simulink model "AGTF30SysLin"  (Simulink 8.5)
settings: Solver=FixedStepDiscrete  StartTime=0.0  StopTime=MWS.In.Max_IterSS  FixedStep=1  RelTol=1e-3
undefined symbols (not defined in the file or in its folder): MWS
libraries: Lib_Cntrl_SetPoint_TMATS x2, Lib_Solve_IterNRSolverJC_TMATS x1, Lib_Solve_Linearize_TMATS x1
settings Model: Creator=jwchapm2  LastModifiedBy=jwchapm2
settings DataIOCC: SignalLoggingSaveFormat=Dataset
settings OptimizationCC: ExpressionDepthLimit=128
settings DebuggingCC: UnderspecifiedInitializationDetection=Simplified  MergeDetectMultiDrivingBlocksExec=error  FcnCallInpInsideContextMsg=EnableAllAsError  StateNameClashWarn=none
settings GRTTargetCC: CombineOutputUpdateFcns=on  GRTInterface=off

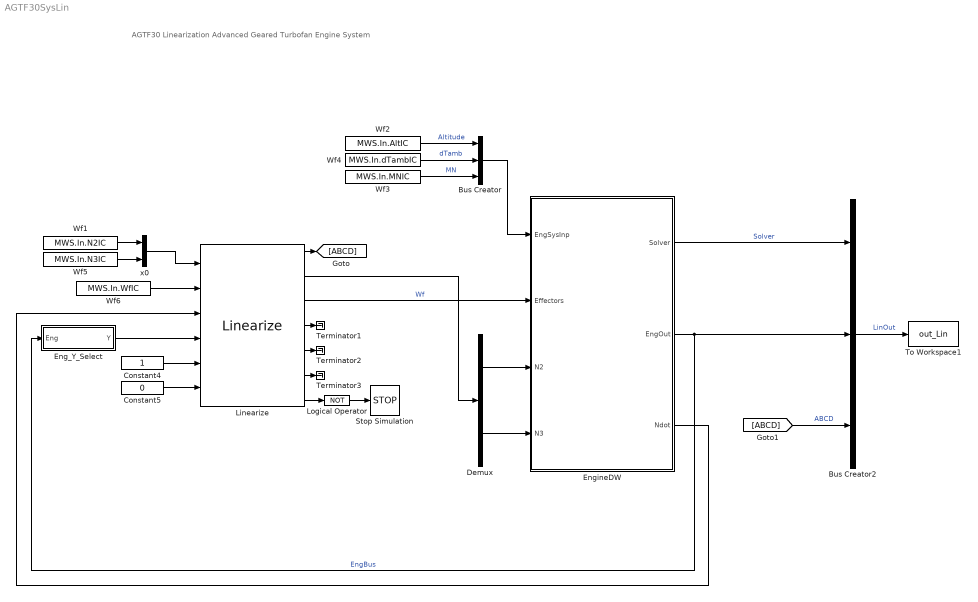
== system AGTF30SysLin ==
  note: AGTF30 Linearization
      | Advanced Geared Turbofan Engine System
  Bus Creator : BusCreator  Inputs=3
  Bus Creator2 : BusCreator  Inputs=3
  Constant4 : Constant
  Constant5 : Constant  Value=0
  Demux : Demux  Outputs=2
  Eng_Y_Select : Subsystem
  EngineDW : Subsystem
  Linearize : Lib_Solve_Linearize_TMATS/Linearize  N_XPer_M=MWS.In.XPerLin  N_UPer_M=MWS.In.UPerLin  N_Y_M=8
  Logical Operator : Logic  Operator=NOT  AllPortsSameDT=off  OutDataTypeStr=boolean
  Stop Simulation : Stop
  Terminator1 : Terminator
  Terminator2 : Terminator
  Terminator3 : Terminator
  To Workspace1 : ToWorkspace  VariableName=out_Lin  SaveFormat=Timeseries  SampleTime=-1
      settings: MaxDataPoints=1
  Wf1 : Constant  Value=MWS.In.N2IC
  Wf2 : Constant  Value=MWS.In.AltIC
  Wf3 : Constant  Value=MWS.In.MNIC
  Wf4 : Constant  Value=MWS.In.dTambIC
  Wf5 : Constant  Value=MWS.In.N3IC
  Wf6 : Constant  Value=MWS.In.WfIC
  x0 : Mux  Inputs=2
  wires:
  Wf2/1 -> Bus Creator/1  "Altitude"
  Wf4/1 -> Bus Creator/2  "dTamb"
  Wf3/1 -> Bus Creator/3  "MN"
  Bus Creator/1 -> EngineDW/1(EngSysInp)
  Demux/1 -> EngineDW/3(N2)
  Demux/2 -> EngineDW/4(N3)
  Linearize/2 -> Demux/1
  Linearize/3 -> EngineDW/2(Effectors)  "Wf"
  Linearize/4 -> Terminator1/1
  Linearize/5 -> Terminator2/1
  Linearize/6 -> Terminator3/1
  Logical Operator/1 -> Stop Simulation/1
  Linearize/7 -> Logical Operator/1
  Constant4/1 -> Linearize/5
  Constant5/1 -> Linearize/6
  Wf1/1 -> x0/1
  Wf5/1 -> x0/2
  x0/1 -> Linearize/1
  Wf6/1 -> Linearize/2
  EngineDW/3(Ndot) -> Linearize/3
  Eng_Y_Select/1(Y) -> Linearize/4
  EngineDW/2(EngOut) -> Eng_Y_Select/1(Eng), Bus Creator2/2  "EngBus"
  EngineDW/1(Solver) -> Bus Creator2/1  "Solver"
  Bus Creator2/1 -> To Workspace1/1  "LinOut"
  Linearize/1 -> [ABCD]
  [ABCD] -> Bus Creator2/3  "ABCD"

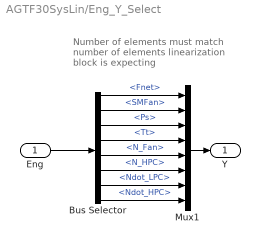
== system AGTF30SysLin/Eng_Y_Select ==
  note: Number of elements must match
      | number of elements linearization
      |  block is expecting
  Eng : Inport
  Bus Selector : BusSelector  OutputSignals=Perf.Fnet,SM.SMFan,S36.Ps,S45.Tt,Shaft.N_Fan,Shaft.N_HPC,Shaft.Ndot_LPC,Shaft.Ndot_HPC
  Mux1 : Mux  Inputs=8
  Y : Outport
  wires:
  Bus Selector/6 -> Mux1/6  "<N_HPC>"
  Bus Selector/5 -> Mux1/5  "<N_Fan>"
  Bus Selector/4 -> Mux1/4  "<Tt>"
  Bus Selector/3 -> Mux1/3  "<Ps>"
  Eng/1 -> Bus Selector/1
  Bus Selector/1 -> Mux1/1  "<Fnet>"
  Mux1/1 -> Y/1
  Bus Selector/2 -> Mux1/2  "<SMFan>"
  Bus Selector/7 -> Mux1/7  "<Ndot_LPC>"
  Bus Selector/8 -> Mux1/8  "<Ndot_HPC>"

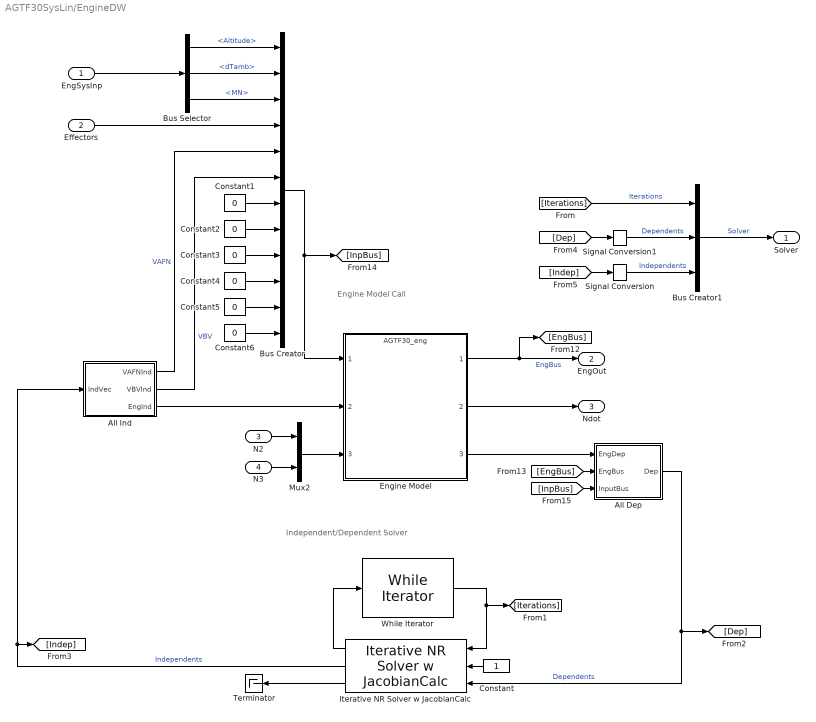
== system AGTF30SysLin/EngineDW ==
  note: Engine Model Call
  note: Independent/Dependent Solver
  EngSysInp : Inport
  Effectors : Inport  Port=2
  N2 : Inport  Port=3
  N3 : Inport  Port=4
  All Dep : Subsystem
  All Ind : Subsystem
  Bus Creator : BusCreator  Inputs=12
  Bus Creator1 : BusCreator  Inputs=3
  Bus Selector : BusSelector  OutputSignals=Altitude,dTamb,MN
  Constant : Constant
  Constant{1..6} (6 alike) : Constant  Value=0
  Engine Model : ModelReference  ModelNameDialog=AGTF30_eng.mdl  SimulationMode=Normal  ModelReferenceVersion=1.312  CopyOfModelName=AGTF30_eng.mdl  DefaultDataLogging=on
  Iterative NR Solver w JacobianCalc : Lib_Solve_IterNRSolverJC_TMATS/Iterative NR Solver w JacobianCalc  SJac_Per_M=[MWS.In.JPerDyn MWS.In.JPerSS(:,10:11)]  SNR_IC_M=[MWS.In.ICcom MWS.In.ICss(4:5)]  SNR_DX_M=MWS.In.dX  SNR_Mx_M=100000  SNR_Mn_M=0.0001  SJacobianAttempts_M=MWS.In.NRASS  Cond_Limits_M=MWS.In.Lim
  Mux2 : Mux  Inputs=2
  Signal Conversion : SignalConversion
  Signal Conversion1 : SignalConversion
  Terminator : Terminator
  While Iterator : WhileIterator  MaxIters=MWS.In.Max_IterSS  WhileBlockType=do-while  ShowIterationPort=on
  Solver : Outport
  EngOut : Outport  Port=2
  Ndot : Outport  Port=3
  wires:
  Signal Conversion1/1 -> Bus Creator1/2  "Dependents"
  Signal Conversion/1 -> Bus Creator1/3  "Independents"
  [Indep] -> Signal Conversion/1
  [Dep] -> Signal Conversion1/1
  Bus Creator1/1 -> Solver/1  "Solver"
  [Iterations] -> Bus Creator1/1  "Iterations"
  Effectors/1 -> Bus Creator/4
  Bus Selector/3 -> Bus Creator/3  "<MN>"
  Bus Selector/2 -> Bus Creator/2  "<dTamb>"
  Bus Selector/1 -> Bus Creator/1  "<Altitude>"
  Engine Model/2 -> Ndot/1
  N3/1 -> Mux2/2
  N2/1 -> Mux2/1
  Iterative NR Solver w JacobianCalc/3 -> Terminator/1
  Mux2/1 -> Engine Model/3
  Iterative NR Solver w JacobianCalc/1 -> While Iterator/1
  While Iterator/1 -> Iterative NR Solver w JacobianCalc/1, [Iterations]
  Iterative NR Solver w JacobianCalc/2 -> All Ind/1(IndVec), [Indep]  "Independents"
  Constant/1 -> Iterative NR Solver w JacobianCalc/2
  EngSysInp/1 -> Bus Selector/1
  Bus Creator/1 -> [InpBus], Engine Model/1
  Engine Model/1 -> [EngBus], EngOut/1  "EngBus"
  All Dep/1(Dep) -> Iterative NR Solver w JacobianCalc/3, [Dep]  "Dependents"
  Engine Model/3 -> All Dep/1(EngDep)
  [EngBus] -> All Dep/2(EngBus)
  [InpBus] -> All Dep/3(InputBus)
  All Ind/1(VAFNInd) -> Bus Creator/5  "VAFN"
  All Ind/2(VBVInd) -> Bus Creator/6  "VBV"
  All Ind/3(EngInd) -> Engine Model/2
  Constant1/1 -> Bus Creator/7
  Constant6/1 -> Bus Creator/12
  Constant5/1 -> Bus Creator/11
  Constant4/1 -> Bus Creator/10
  Constant3/1 -> Bus Creator/9
  Constant2/1 -> Bus Creator/8

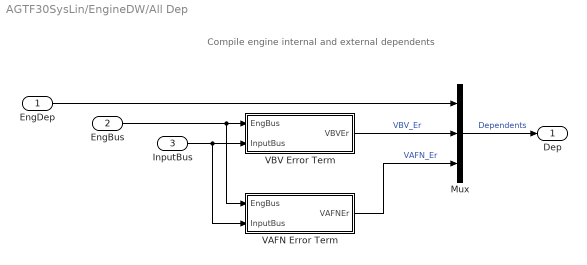
== system AGTF30SysLin/EngineDW/All Dep ==
  note: Compile engine internal and external dependents
  EngDep : Inport
  EngBus : Inport  Port=2
  InputBus : Inport  Port=3
  Mux : Mux  Inputs=3
  VAFN Error Term : Subsystem
  VBV Error Term : Subsystem
  Dep : Outport
  wires:
  EngBus/1 -> VAFN Error Term/1(EngBus), VBV Error Term/1(EngBus)
  Mux/1 -> Dep/1  "Dependents"
  VBV Error Term/1(VBVEr) -> Mux/2  "VBV_Er"
  EngDep/1 -> Mux/1
  VAFN Error Term/1(VAFNEr) -> Mux/3  "VAFN_Er"
  InputBus/1 -> VAFN Error Term/2(InputBus), VBV Error Term/2(InputBus)

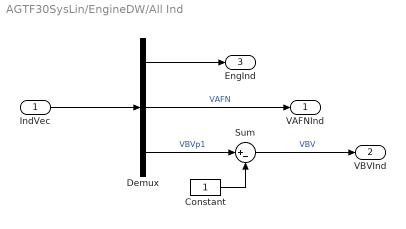
== system AGTF30SysLin/EngineDW/All Ind ==
  IndVec : Inport
  Constant : Constant
  Demux : Demux  Outputs=[7 1 1]
  Sum : Sum  Inputs=|+-
  VAFNInd : Outport
  VBVInd : Outport  Port=2
  EngInd : Outport  Port=3
  wires:
  Demux/1 -> EngInd/1
  IndVec/1 -> Demux/1
  Demux/3 -> Sum/1  "VBVp1"
  Demux/2 -> VAFNInd/1  "VAFN"
  Sum/1 -> VBVInd/1  "VBV"
  Constant/1 -> Sum/2

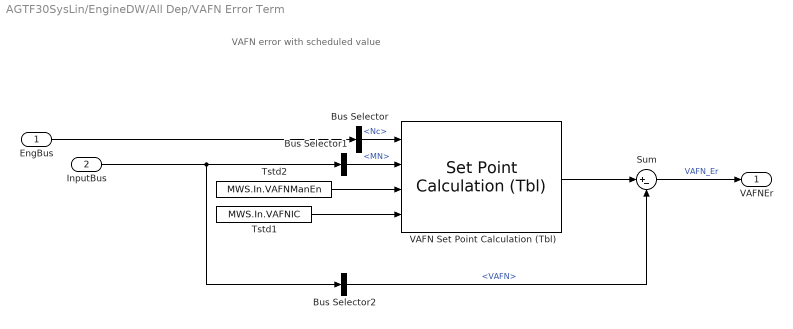
== system AGTF30SysLin/EngineDW/All Dep/VAFN Error Term ==
  note: VAFN error with scheduled value
  EngBus : Inport
  InputBus : Inport  Port=2
  Bus Selector : BusSelector  OutputSignals=Data.FAN_Data.Nc
  Bus Selector1 : BusSelector  OutputSignals=MN
  Bus Selector2 : BusSelector  OutputSignals=VAFN
  Sum : Sum  Inputs=|+-
  Tstd1 : Constant  Value=MWS.In.VAFNIC
  Tstd2 : Constant  Value=MWS.In.VAFNManEn
  VAFN Set Point Calculation (Tbl) : Lib_Cntrl_SetPoint_TMATS/Set Point Calculation (Tbl)  ERVec_M=MWS.Cntrl.VAFN_Nc1  DSVec_M=MWS.Cntrl.VAFN_MN  SPArray_M=MWS.Cntrl.VAFN_sch
  VAFNEr : Outport
  wires:
  Bus Selector1/1 -> VAFN Set Point Calculation (Tbl)/2  "<MN>"
  EngBus/1 -> Bus Selector/1
  VAFN Set Point Calculation (Tbl)/1 -> Sum/1
  Tstd2/1 -> VAFN Set Point Calculation (Tbl)/3
  Tstd1/1 -> VAFN Set Point Calculation (Tbl)/4
  Bus Selector/1 -> VAFN Set Point Calculation (Tbl)/1  "<Nc>"
  Sum/1 -> VAFNEr/1  "VAFN_Er"
  InputBus/1 -> Bus Selector2/1, Bus Selector1/1
  Bus Selector2/1 -> Sum/2  "<VAFN>"

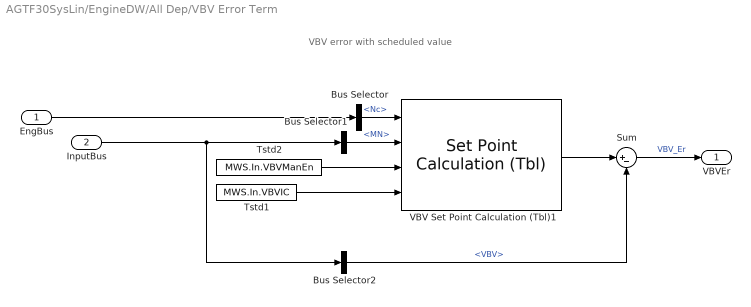
== system AGTF30SysLin/EngineDW/All Dep/VBV Error Term ==
  note: VBV error with scheduled value
  EngBus : Inport
  InputBus : Inport  Port=2
  Bus Selector : BusSelector  OutputSignals=Data.FAN_Data.Nc
  Bus Selector1 : BusSelector  OutputSignals=MN
  Bus Selector2 : BusSelector  OutputSignals=VBV
  Sum : Sum  Inputs=|+-
  Tstd1 : Constant  Value=MWS.In.VBVIC
  Tstd2 : Constant  Value=MWS.In.VBVManEn
  VBV Set Point Calculation (Tbl)1 : Lib_Cntrl_SetPoint_TMATS/Set Point Calculation (Tbl)  ERVec_M=MWS.Cntrl.VBV_Nc1  DSVec_M=MWS.Cntrl.VBV_MN  SPArray_M=MWS.Cntrl.VBV_sch
  VBVEr : Outport
  wires:
  Bus Selector2/1 -> Sum/2  "<VBV>"
  InputBus/1 -> Bus Selector1/1, Bus Selector2/1
  Sum/1 -> VBVEr/1  "VBV_Er"
  Bus Selector/1 -> VBV Set Point Calculation (Tbl)1/1  "<Nc>"
  Tstd1/1 -> VBV Set Point Calculation (Tbl)1/4
  Tstd2/1 -> VBV Set Point Calculation (Tbl)1/3
  VBV Set Point Calculation (Tbl)1/1 -> Sum/1
  EngBus/1 -> Bus Selector/1
  Bus Selector1/1 -> VBV Set Point Calculation (Tbl)1/2  "<MN>"
